simulink model "lab63"  (R2023b)
settings: Solver=VariableStepAuto  StartTime=0.0  StopTime=50  RelTol=1e-3
model workspace (MAT data in the model file):
  kp_PWM = 0.0200507272725
libraries: checkpacklib x1
settings Model: Creator=Настя  LastModifiedBy=killer
settings SolverCC: AlgebraicLoopSolver=TrustRegion
settings DebuggingCC: UnconnectedInputMsg=warning  UnconnectedOutputMsg=warning  UnconnectedLineMsg=warning
settings ModelReferenceCC: EnableRefExpFcnMdlSchedulingChecks=on
settings RTWCC: DLArmComputeVersion=19.05

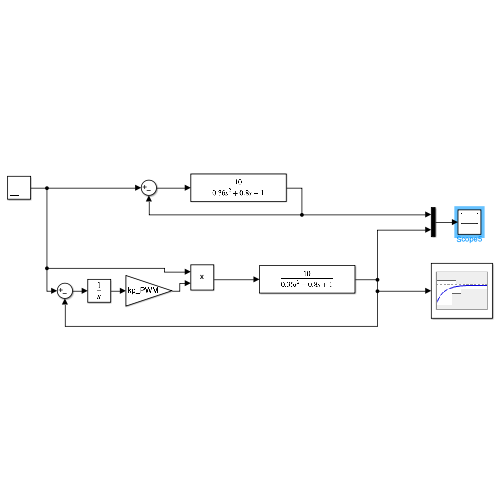
[thumbnail: Simulink's stored preview of the top-level diagram]
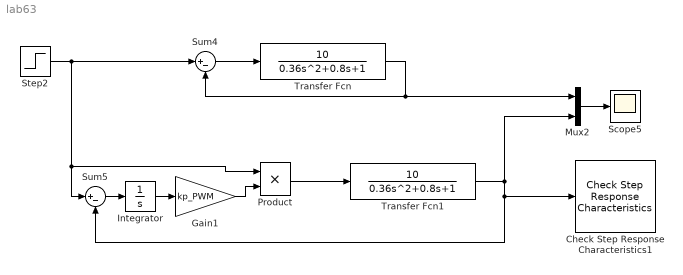
== system lab63 ==
  Check Step Response Characteristics1 : checkpacklib/Check Step Response  Characteristics  InstantiateOnLoad=on  enabled=on  stopWhenAssertionFail=off  export=off  ViewDlgPos=[]  OpenViewOnLoad=off  LaunchViewOnOpen=off  TimeUnits=seconds  EnableStepResponseBound=on  InitialValue=0  FinalValue=1  StepTime=0  RiseTime=5  PercentRise=80  SettlingTime=7  PercentSettling=1  PercentOvershoot=10  PercentUndershoot=1
  Gain1 : Gain  Gain=kp_PWM
  Integrator : Integrator
  Mux2 : Mux  Inputs=2
  Product : Product
  Scope5 : Scope
  Step2 : Step  Time=0  SampleTime=0
  Sum4 : Sum  Inputs=|+-
  Sum5 : Sum  Inputs=|+-
  Transfer Fcn : TransferFcn  Numerator=[10]  Denominator=[0.36 0.8 1]
  Transfer Fcn1 : TransferFcn  Numerator=[10]  Denominator=[0.36 0.8 1]
  wires:
  Transfer Fcn1/1 -> Sum5/2, Check Step Response Characteristics1/1, Mux2/2
  Sum5/1 -> Integrator/1
  Gain1/1 -> Product/2
  Product/1 -> Transfer Fcn1/1
  Integrator/1 -> Gain1/1
  Step2/1 -> Product/1, Sum5/1, Sum4/1
  Sum4/1 -> Transfer Fcn/1
  Mux2/1 -> Scope5/1
  Transfer Fcn/1 -> Sum4/2, Mux2/1
